simulink library "sadc_library_old"  (R2020b)
settings: Solver=VariableStepAuto  StartTime=0.0  StopTime=10.0  RelTol=1e-3
undefined symbols (not defined in the file): actuators, constants, control, magnitude, orbit, sensors
libraries: vrlib x12
(part 2 of 2)

== matlab function sadc_library_old/Environment/Solar radiation pressure/MATLAB Function ==
  data: mjd2000 input; kep output
function  kep = uplanet(mjd2000)

% uplanet.m - Analytical ephemerides for planets
%
% PROTOTYPE:
%  [kep, ksun] = uplanet (mjd2000, ibody);
%
% DESCRIPTION:
%   Planetary orbital elements are restituited in a Sun-centred ecliptic 
%   system.
%   These ephemerides were succesfully compared with JPL/NAIF/SPICE
%   ephemerides using de405.bps.
%
%  INPUT :
%	mjd2000[1]  Time, modified Julian day since 01/01/2000, 12:00 noon
%               (MJD2000 = MJD-51544.5)
%	ibody[1]    Integer number identifying the celestial body (< 11)
%                   1:   Mercury
%                   2:   Venus
%                   3:   Earth
%                   4:   Mars
%                   5:   Jupiter
%                   6:   Saturn
%                   7:   Uranus
%                   8:   Neptune
%                   9:   Pluto
%                   10:  Sun
%
%  OUTPUT:
%	kep[6]    	Mean Keplerian elements of date
%                 kep = [a e i Om om theta] [km, rad]
%	ksun[1]     Gravity constant of the Sun [km^3/s^2]
%
%   Note: The ephemerides of the Moon are given by EphSS_kep, according to
%           to the algorithm in ephMoon.m
%
%  FUNCTIONS CALLED:
%   (none)
%
% AUTHOR:
%   P. Dysli, 1977
%
% PREVIOUS VERSION:
%   P. Dysli, 1977, MATLAB, uplanet.m
%       - Header and function name in accordance with guidlines.
%
%  CHANGELOG:
%   28/12/06, Camilla Colombo: tidied up
%   10/01/2007, REVISION, Matteo Ceriotti 
%   03/05/2008, Camilla Colombo: Case 11 deleted.
%   11/09/2008, Matteo Ceriotti, Camilla Colombo:
%       - All ephemerides shifted 0.5 days back in time. Now mjd2000 used
%           in this function is referred to 01/01/2000 12:00. In the old
%           version it was referred to 02/01/2000 00:00.
%       - Corrected ephemeris of Pluto.
%   04/10/2010, Camilla Colombo: Header and function name in accordance
%       with guidlines.
%
% -------------------------------------------------------------------------

DEG2RAD=pi/180;

G=6.67259e-20;
msun=1.988919445342813e+030;
kep = zeros(6,1);
KM  = 149597870.66;

%  T = JULIAN CENTURIES SINCE 31/12/1899 at 12:00
T   = (mjd2000 + 36525)/36525.00;
TT  = T*T;
TTT = T*TT;
kep(1)=T*0;

%
%  CLASSICAL PLANETARY ELEMENTS ESTIMATION IN MEAN ECLIPTIC OF DATE
%

    %  EARTH
    %
        kep(1) = 1.000000230;
        kep(2) = 0.016751040 - 0.000041800*T - 0.0000001260*TT;
        kep(3) = 0.00;
    	kep(4) = 0.00;
      	kep(5) = 1.01220833333333333e+2 + 1.7191750*T + 4.52777777777777778e-4*TT + 3.33333333333333333e-6*TTT;
     	XM   = 3.599904975e+4 - 1.50277777777777778e-4*T - 3.33333333333333333e-6*TT;
     	kep(6) = 3.58475844444444444e2 + XM*T;

  
%
%  CONVERSION OF AU INTO KM, DEG INTO RAD AND DEFINITION OF  XMU
%
 
kep(1)   = kep(1)*KM;       % a [km]
kep(3:6) = kep(3:6)*DEG2RAD;    % Transform from deg to rad
kep(6)   = mod(kep(6),2*pi);
% XMU  = (XM*DEG2RAD/(864000*365250))^2*kep(1)^3;
phi    = kep(6);          % phi is the eccentric anomaly, uses kep(6)=M as a first guess
     
for i=1:5
    g       = kep(6)-(phi-kep(2)*sin(phi)); 
	g_primo = (-1+kep(2)*cos(phi));
 	phi     = phi-g/g_primo;   % Computes the eccentric anomaly kep
end 

theta=2*atan(sqrt((1+kep(2))/(1-kep(2)))*tan(phi/2));

kep(6)=theta;

return

== matlab function sadc_library_old/Environment/Solar radiation pressure/MATLAB Function1 ==
  data: kep input; rr output
function rr = kep2car(kep)
% 
% Function to compute position and velocity vectors of the satellite the 
% keplerian elements.
% 
% INPUT:
%  a [1]       Semimajor axis [km]
%  e [1]       Eccentricity [-]
%  i [1]       Inclination angle [rad]
%  OM [1]      Right ascention of the ascending node [rad]
%  om [1]      Anomaly of the pericenter [rad]
%  th [1]      True anomaly [rad]
%  MU [1]      Gravitational parameter of the primary [km^3/s^2]
% 
% OUTPUT:
%  rr [3,1]    Position vector in inertial frame [km]
%  vv [3,1]    Velocity vector in inertial frame [km/s]
% 
a = kep(1); e = kep(2); i = kep(3); OM = kep(4); om = kep(5); theta = kep(6);

p = a*(1-e^2);
r = p/(1+e*cos(theta));

rr = r*[cos(theta);sin(theta);0];

ROM = [ cos(OM) sin(OM) 0; -sin(OM) cos(OM) 0; 0 0 1];
Ri = [ 1 0 0; 0 cos(i) sin(i); 0 -sin(i) cos(i)];
Rom = [ cos(om) sin(om) 0; -sin(om) cos(om) 0; 0 0 1];

T = Rom*Ri*ROM;

rr = T'*rr;

end

== matlab function sadc_library_old/Environment/Solar radiation pressure/MATLAB Function2 ==
  data: rr input; shadow_cone output; rr_sun_eq input
function shadow_cone = cone(rr, rr_sun_eq)

% PROTOTYPE:
%  shadow_cone = cone(rr_sc, rr_sun)
% 
% DESCRIPTION:
%   This function returns a parameter that is 1 if the s/c is out of the 
%   planet's shadow cone (SRP effects considerable) or 0 if the s/c is 
%   inside the planet's shadow cone (NO SRP)
% 
% INPUT:
% rr_sc:            geocentric position vector of the s/c
% rr_sun_eq:        geocentric position vector of the sun
%
% OUTPUT:
% shadow_cone:      boolean parameter (0 or 1)
%
% CONTRIBUTORS:
% Velo Giacomo
%
% VERSIONS:
% 2019-12-10 first version
%
% CALLED FUNCTIONS:
%     none


R_e = 6378.137;
r_sc = norm(rr);     
r_sun = norm(rr_sun_eq);
% Angle between s/c geocentric position and the tangent to Earth's surface
theta_sc = acos(R_e/r_sc);
% Angle between sun geocentric position and the tangent to Earth's surface
theta_sun = acos(R_e/r_sun);
% Angle between s/c geocentric position and sun geocentric position
theta = acos(dot(rr, rr_sun_eq)/(r_sc*r_sun));

% If the s/c is inside the shadow cone of the planet the value of
% shadow_cone will be = 0

    if theta_sc + theta_sun <= theta
        shadow_cone = 0;
    else
        shadow_cone = 1;
    end

end

== matlab function sadc_library_old/Kinematics/Quaternion integration/MATLAB Function ==
  data: w input; OM_mat output
function OM_mat = quat_matrix(w)

wx = w(1);
wy = w(2);
wz = w(3);

OM_mat = [0, wz, -wy, wx;...
    -wx, 0, wx, wy;...
    wy, -wx, 0, wz;...
    -wx, -wy, -wz, 0];
    
end

== matlab function sadc_library_old/Orbit propagator/MATLAB Function4 ==
  data: a_J2 output; rr input
function a_J2 = J2_perturb(rr)

J2 = 0.00108263;
Req = 6378.1;
mu_e = 398600;

r = norm(rr);
rx = rr(1);
ry = rr(2);
rz = rr(3);

a_J2 = 3/2*J2*mu_e*Req^2/(r^4)*[rx/r*(5*(rz/r)^2 - 1);...
    ry/r*(5*(rz/r)^2 - 1);...
    rz/r*(5*(rz/r)^2 - 3)];

end

== matlab function sadc_library_old/Orbit propagator/MATLAB Function5 ==
  data: rr input; kep output; vv input
function kep = car2kep(rr, vv)

mu_e = 398600;

r = norm(rr);
v = norm(vv);

hh = cross(rr,vv);
h = norm(hh);
i = acos(hh(3)/h);

a = -mu_e/2*1/(v^2/2 - mu_e/r);

k = [0 0 1];
nn = cross(k,hh);
nn = nn/norm(nn);

if nn(2) < 0
    OM = 2*pi - acos(nn(1));
else
    OM = acos(nn(1));
end

ee = cross(vv,hh)/mu_e - rr/r;
e = norm(ee);

if ee(3) < 0
    om = 2*pi - acos(dot(nn,ee)/e);
else
    om = acos(dot(nn,ee)/e);
end

vr = dot(rr,vv);

if vr < 0
    theta = 2*pi - acos(dot(rr,ee)/r/e);
else
    theta = acos(dot(rr,ee)/r/e);
end

kep = [a; e; i; OM; om; theta];

end

== matlab function sadc_library_old/Environment/Solar radiation pressure/If Action Subsystem1/MATLAB Function ==
  data: s_b input; P input; Fsrp_b output; Msrp output; surfaces parameter
function [Fsrp_b, Msrp] = srp(s_b, P, surfaces)

rhoS_body = surfaces.body.rhoS;
rhoD_body = surfaces.body.rhoD;

rhoS_panels = surfaces.panels.rhoS;
rhoD_panels = surfaces.panels.rhoD;

nf_body = surfaces.body.num;
nf_panels = surfaces.panels.num;

r_surf_body = surfaces.body.r_surf;
r_surf_panels = surfaces.panels.r_surf;
n_body = surfaces.body.n;
n_panels = surfaces.panels.n;

A_body = surfaces.body.A;
A_panels = surfaces.panels.A;

Fsrp_b = zeros(3,1);
Msrp = zeros(3,1);

for k = 1:nf_panels
    n_b = n_panels(k,:)';
    s_dot = dot(s_b, n_b);
    if s_dot > 0
        Fsrp_i = - P*A_panels(k)*s_dot.*((1-rhoS_panels).*s_b +...
            (2*rhoS_panels*s_dot + 2/3*rhoD_panels).*n_b);
        Fsrp_b = Fsrp_b + Fsrp_i;
        Msrp = Msrp + cross(r_surf_panels(k,:)', Fsrp_i);
    end
end

for k = 1:nf_body
    n_b = n_body(k,:)';
    s_dot = dot(s_b, n_b);
    if s_dot > 0
        Fsrp_i = - P*A_body(k)*s_dot.*((1-rhoS_body).*s_b +...
            (2*rhoS_body*s_dot + 2/3*rhoD_body).*n_b);
        Fsrp_b = Fsrp_b + Fsrp_i;
        Msrp = Msrp + cross(r_surf_body(k,:)', Fsrp_i);
    end
end

% aggiungere questione su "ombra aerodinamica"

end

== matlab function sadc_library_old/Environment/Gravity gradient torque/MATLAB Function1 ==
  data: theta input; A_li output
function A_li = inclined_to_orbital(theta)

A_li = [cos(theta), sin(theta), 0;...
    -sin(theta), cos(theta), 0;...
    0, 0, 1];

end
